simulink library "halin"  (R2021b)
settings: Solver=VariableStepAuto  StartTime=0.0  StopTime=10.0  RelTol=1e-3
undefined symbols (not defined in the file): TRUE
libraries: FVT_lib x100, hcu_lib x41
(part 1 of 10)
settings Model: Creator=13168  LastModifiedBy=FVT23010
settings SolverCC: AlgebraicLoopSolver=TrustRegion
settings DataIOCC: SaveFormat=Array  SignalLoggingSaveFormat=ModelDataLogs  ReturnWorkspaceOutputs=off
settings OptimizationCC: BlockReduction=off  BooleanDataType=off
settings DebuggingCC: SaveWithParameterizedLinksMsg=none  UnderspecifiedInitializationDetection=Classic  MergeDetectMultiDrivingBlocksExec=none  SignalResolutionControl=TryResolveAllWithWarning  SFMachineParentedDataDiag=warning
settings HardwareCC: TargetUnknown=on
settings ModelReferenceCC: PropagateSignalLabelsOutOfModel=off
settings ConfigComp: CovMetricSettings=dw  CovSaveCumulativeToWorkspaceVar=on  CovSaveSingleToWorkspaceVar=on

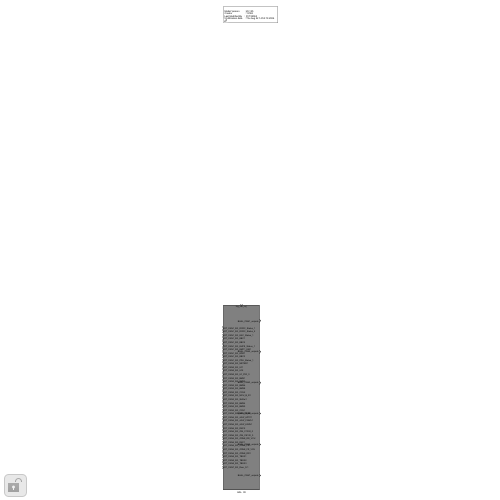
[thumbnail: Simulink's stored preview of the top-level diagram]
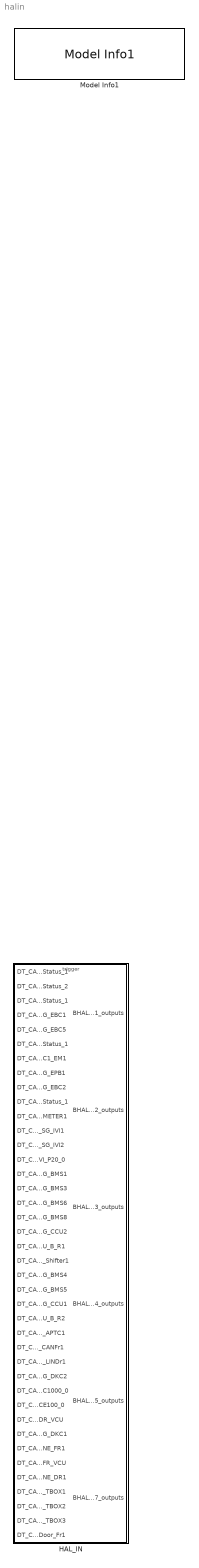
== system halin ==
  HAL_IN : Subsystem
      settings: RTWSystemCode=Nonreusable function  RTWFcnNameOpts=Use subsystem name  RTWFileNameOpts=Use subsystem name
  Model Info1 : hcu_lib/Model Info1  BlockCM=None  Frame=on  DisplayStringWithTags=|  HorizontalTextAlignment=Left  LeftAlignmentValue=0.02  SourceBlockDiagram=hcu_lib  TagMaxNumber=20
      | Model Version        : %<ModelVersion>
      | Creator                   : %<Creator>
      | Last Modified By    : %<LastModifiedBy>
      | Modification date    : %<LastModificationDate>
      settings: SourceProductName=HCU Relative Block Library

== system halin/HAL_IN ==
  DT_CAN1_SG_DCDC_Status_1 : Inport
  DT_CAN1_SG_DCDC_Status_2 : Inport  Port=2
  DT_CAN1_SG_EAC_Status_1 : Inport  Port=3
  DT_CAN1_SG_EBC1 : Inport  Port=4
  DT_CAN1_SG_EBC5 : Inport  Port=5
  DT_CAN1_SG_EHPS_Status_1 : Inport  Port=6
  DT_CAN1_SG_EMC1_EM1 : Inport  Port=7
  DT_CAN1_SG_EPB1 : Inport  Port=8
  DT_CAN1_SG_EBC2 : Inport  Port=9
  DT_CAN1_SG_PDU_Status_1 : Inport  Port=10
  DT_CAN2_SG_METER1 : Inport  Port=11
  DT_CAN2_SG_IVI1 : Inport  Port=12
  DT_CAN2_SG_IVI2 : Inport  Port=13
  DT_CAN2_SG_IVI_P20_0 : Inport  Port=14
  DT_CAN3_SG_BMS1 : Inport  Port=15
  DT_CAN3_SG_BMS3 : Inport  Port=16
  DT_CAN3_SG_BMS6 : Inport  Port=17
  DT_CAN3_SG_BMS8 : Inport  Port=18
  DT_CAN3_SG_CCU2 : Inport  Port=19
  DT_CAN3_SG_MCU_B_R1 : Inport  Port=20
  DT_CAN3_SG_Shifter1 : Inport  Port=21
  DT_CAN3_SG_BMS4 : Inport  Port=22
  DT_CAN3_SG_BMS5 : Inport  Port=23
  DT_CAN3_SG_CCU1 : Inport  Port=24
  DT_CAN3_SG_MCU_B_R2 : Inport  Port=25
  DT_CAN4_SG_zGW_APTC1 : Inport  Port=26
  DT_CAN4_SG_zGW_CANFr1 : Inport  Port=27
  DT_CAN4_SG_zGW_LINDr1 : Inport  Port=28
  DT_CAN4_SG_DKC2 : Inport  Port=29
  DT_CAN4_SG_Z24_C1000_0 : Inport  Port=30
  DT_CAN4_SG_Z24_CE100_0 : Inport  Port=31
  DT_CAN4_SG_ZONE_DR_VCU : Inport  Port=32
  DT_CAN4_SG_DKC1 : Inport  Port=33
  DT_CAN4_SG_ZONE_FR1 : Inport  Port=34
  DT_CAN4_SG_ZONE_FR_VCU : Inport  Port=35
  DT_CAN4_SG_ZONE_DR1 : Inport  Port=36
  DT_CAN5_SG_TBOX1 : Inport  Port=37
  DT_CAN5_SG_TBOX2 : Inport  Port=38
  DT_CAN5_SG_TBOX3 : Inport  Port=39
  DT_CAN7_SG_Door_Fr1 : Inport  Port=40
  trig_hal_in : TriggerPort  TriggerType=function-call  VariantControl=(inherit)
  CAN1 : Subsystem
  CAN2 : Subsystem
  CAN3 : Subsystem
  CAN4 : Subsystem
  CAN5 : Subsystem
  CAN7 : Subsystem
  BHAL_CAN1_outputs : Outport  OutDataTypeStr=Bus: BHAL_CAN1_outputs
  BHAL_CAN2_outputs : Outport  Port=2  OutDataTypeStr=Bus: BHAL_CAN2_outputs
  BHAL_CAN3_outputs : Outport  Port=3  OutDataTypeStr=Bus: BHAL_CAN3_outputs
  BHAL_CAN4_outputs : Outport  Port=4  OutDataTypeStr=Bus: BHAL_CAN4_outputs
  BHAL_CAN5_outputs : Outport  Port=5  OutDataTypeStr=Bus: BHAL_CAN5_outputs
  BHAL_CAN7_outputs : Outport  Port=6  OutDataTypeStr=Bus: BHAL_CAN7_outputs
  wires:
  DT_CAN5_SG_TBOX1/1 -> CAN5/1(DT_CAN5_SG_TBOX1)
  DT_CAN3_SG_CCU1/1 -> CAN3/10(DT_CAN3_SG_CCU1)
  DT_CAN3_SG_BMS5/1 -> CAN3/9(DT_CAN3_SG_BMS5)
  DT_CAN3_SG_BMS4/1 -> CAN3/8(DT_CAN3_SG_BMS4)
  DT_CAN3_SG_Shifter1/1 -> CAN3/7(DT_CAN3_SG_Shifter1)
  DT_CAN3_SG_MCU_B_R1/1 -> CAN3/6(DT_CAN3_SG_MCU_B_R1)
  DT_CAN3_SG_CCU2/1 -> CAN3/5(DT_CAN3_SG_CCU2)
  DT_CAN3_SG_BMS8/1 -> CAN3/4(DT_CAN3_SG_BMS8)
  CAN7/1(HAL_CAN7_outputs) -> BHAL_CAN7_outputs/1
  DT_CAN3_SG_BMS3/1 -> CAN3/2(DT_CAN3_SG_BMS3)
  DT_CAN3_SG_BMS1/1 -> CAN3/1(DT_CAN3_SG_BMS1)
  CAN1/1(HAL_CAN1_outputs) -> BHAL_CAN1_outputs/1
  CAN3/1(HAL_CAN3_outputs) -> BHAL_CAN3_outputs/1
  CAN4/1(HAL_CAN4_outputs) -> BHAL_CAN4_outputs/1
  DT_CAN1_SG_EMC1_EM1/1 -> CAN1/7(DT_CAN1_SG_EMC1_EM1)
  DT_CAN1_SG_EBC5/1 -> CAN1/5(DT_CAN1_SG_EBC5)
  DT_CAN1_SG_EHPS_Status_1/1 -> CAN1/6(DT_CAN1_SG_EHPS_Status_1)
  DT_CAN1_SG_EBC1/1 -> CAN1/4(DT_CAN1_SG_EBC1)
  DT_CAN1_SG_EAC_Status_1/1 -> CAN1/3(DT_CAN1_SG_EAC_Status_1)
  DT_CAN3_SG_BMS6/1 -> CAN3/3(DT_CAN3_SG_BMS6)
  DT_CAN1_SG_DCDC_Status_2/1 -> CAN1/2(DT_CAN1_SG_DCDC_Status_2)
  DT_CAN4_SG_ZONE_DR1/1 -> CAN4/11(DT_CAN4_SG_ZONE_DR1)
  DT_CAN1_SG_DCDC_Status_1/1 -> CAN1/1(DT_CAN1_SG_DCDC_Status_1)
  CAN2/1(HAL_CAN2_outputs) -> BHAL_CAN2_outputs/1
  DT_CAN3_SG_MCU_B_R2/1 -> CAN3/11(DT_CAN3_SG_MCU_B_R2)
  DT_CAN2_SG_IVI1/1 -> CAN2/2(DT_CAN2_SG_IVI1)
  DT_CAN5_SG_TBOX3/1 -> CAN5/3(DT_CAN5_SG_TBOX3)
  DT_CAN2_SG_METER1/1 -> CAN2/1(DT_CAN2_SG_METER1)
  DT_CAN1_SG_PDU_Status_1/1 -> CAN1/10(DT_CAN1_SG_PDU_Status_1)
  DT_CAN7_SG_Door_Fr1/1 -> CAN7/1(DT_CAN7_SG_Door_Fr1)
  DT_CAN1_SG_EPB1/1 -> CAN1/8(DT_CAN1_SG_EPB1)
  DT_CAN1_SG_EBC2/1 -> CAN1/9(DT_CAN1_SG_EBC2)
  DT_CAN2_SG_IVI2/1 -> CAN2/3(DT_CAN2_SG_IVI2)
  DT_CAN5_SG_TBOX2/1 -> CAN5/2(DT_CAN5_SG_TBOX2)
  DT_CAN2_SG_IVI_P20_0/1 -> CAN2/4(DT_CAN2_SG_IVI_P20_0)
  CAN5/1(HAL_CAN5_outputs) -> BHAL_CAN5_outputs/1
  DT_CAN4_SG_DKC1/1 -> CAN4/1(DT_CAN4_SG_DKC1)
  DT_CAN4_SG_ZONE_DR_VCU/1 -> CAN4/2(DT_CAN4_SG_ZONE_DR_VCU)
  DT_CAN4_SG_ZONE_FR1/1 -> CAN4/3(DT_CAN4_SG_ZONE_FR1)
  DT_CAN4_SG_ZONE_FR_VCU/1 -> CAN4/4(DT_CAN4_SG_ZONE_FR_VCU)
  DT_CAN4_SG_zGW_APTC1/1 -> CAN4/5(DT_CAN4_SG_zGW_APTC1)
  DT_CAN4_SG_zGW_LINDr1/1 -> CAN4/7(DT_CAN4_SG_zGW_LINDr1)
  DT_CAN4_SG_DKC2/1 -> CAN4/8(DT_CAN4_SG_DKC2)
  DT_CAN4_SG_Z24_C1000_0/1 -> CAN4/9(DT_CAN4_SG_Z24_C1000_0)
  DT_CAN4_SG_Z24_CE100_0/1 -> CAN4/10(DT_CAN4_SG_Z24_CE100_0)
  DT_CAN4_SG_zGW_CANFr1/1 -> CAN4/6(DT_CAN4_SG_zGW_CANFr1)

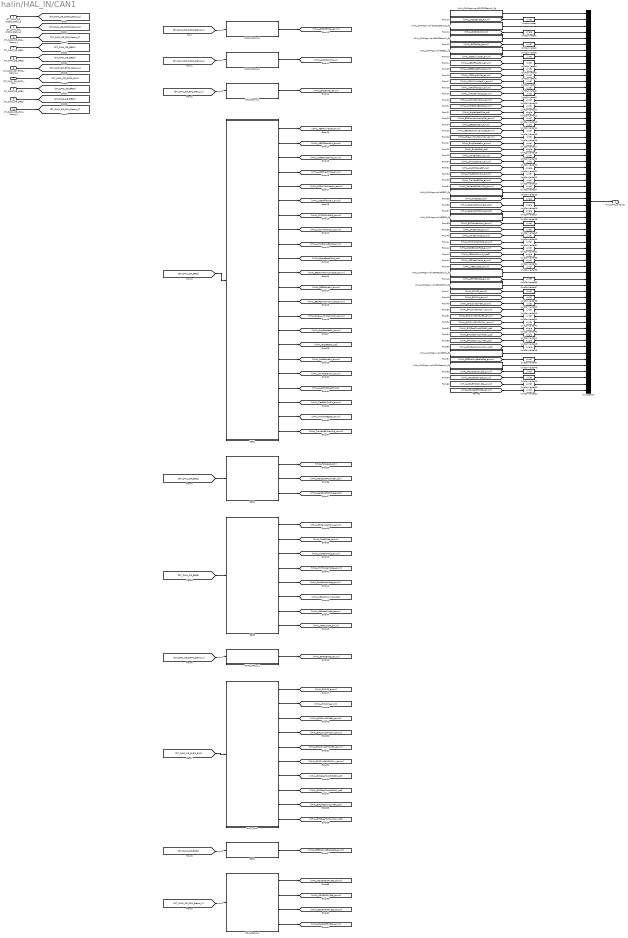
== system halin/HAL_IN/CAN1 ==
  DT_CAN1_SG_DCDC_Status_1 : Inport
  DT_CAN1_SG_DCDC_Status_2 : Inport  Port=2
  DT_CAN1_SG_EAC_Status_1 : Inport  Port=3
  DT_CAN1_SG_EBC1 : Inport  Port=4
  DT_CAN1_SG_EBC5 : Inport  Port=5
  DT_CAN1_SG_EHPS_Status_1 : Inport  Port=6
  DT_CAN1_SG_EMC1_EM1 : Inport  Port=7
  DT_CAN1_SG_EPB1 : Inport  Port=8
  DT_CAN1_SG_EBC2 : Inport  Port=9
  DT_CAN1_SG_PDU_Status_1 : Inport  Port=10
  DCDC_Status_1 : Subsystem
  DCDC_Status_2 : Subsystem
  EAC_Status_1 : Subsystem
  EBC1 : Subsystem
  EBC2 : Subsystem
  EBC5 : Subsystem
  EHPS_Status_1 : Subsystem
  EMC1_EM1 : Subsystem
  EPB1 : Subsystem
  PDU_Status_1 : Subsystem
  UnitConverter{,2..11,13..17,19..20,22..24,28..32,34..42,47..51} (40 alike) : DataTypeConversion  OutDataTypeStr=uint8
  UnitConverter{1,12,18,21,25..27,33,43..46} (12 alike) : DataTypeConversion  OutDataTypeStr=single
  VHAL_CANMsgInvalidDCDCStatus1_flg : Subsystem  AncestorBlock=FVT_lib/hal/MsgTimeoutJudge_CAN_AUTOSAR
      mask help: MeasumentTrigerEvent
      mask Display: fprintf('MsgTimeoutJudge_CAN\nAUTOSAR');
  VHAL_CANMsgInvalidDCDCStatus2_flg : Subsystem  AncestorBlock=FVT_lib/hal/MsgTimeoutJudge_CAN_AUTOSAR
      mask help: MeasumentTrigerEvent
      mask Display: fprintf('MsgTimeoutJudge_CAN\nAUTOSAR');
  VHAL_CANMsgInvalidEACStatus1_flg : Subsystem  AncestorBlock=FVT_lib/hal/MsgTimeoutJudge_CAN_AUTOSAR
      mask help: MeasumentTrigerEvent
      mask Display: fprintf('MsgTimeoutJudge_CAN\nAUTOSAR');
  VHAL_CANMsgInvalidEBC1_flg : Subsystem  AncestorBlock=FVT_lib/hal/MsgTimeoutJudge_CAN_AUTOSAR
      mask help: MeasumentTrigerEvent
      mask Display: fprintf('MsgTimeoutJudge_CAN\nAUTOSAR');
  VHAL_CANMsgInvalidEBC2_flg : Subsystem  AncestorBlock=FVT_lib/hal/MsgTimeoutJudge_CAN_AUTOSAR
      mask help: MeasumentTrigerEvent
      mask Display: fprintf('MsgTimeoutJudge_CAN\nAUTOSAR');
  VHAL_CANMsgInvalidEBC5_flg : Subsystem  AncestorBlock=FVT_lib/hal/MsgTimeoutJudge_CAN_AUTOSAR
      mask help: MeasumentTrigerEvent
      mask Display: fprintf('MsgTimeoutJudge_CAN\nAUTOSAR');
  VHAL_CANMsgInvalidEHPSStatus1_flg : Subsystem  AncestorBlock=FVT_lib/hal/MsgTimeoutJudge_CAN_AUTOSAR
      mask help: MeasumentTrigerEvent
      mask Display: fprintf('MsgTimeoutJudge_CAN\nAUTOSAR');
  VHAL_CANMsgInvalidEMC1EM1_flg : Subsystem  AncestorBlock=FVT_lib/hal/MsgTimeoutJudge_CAN_AUTOSAR
      mask help: MeasumentTrigerEvent
      mask Display: fprintf('MsgTimeoutJudge_CAN\nAUTOSAR');
  VHAL_CANMsgInvalidEPB1_flg : Subsystem  AncestorBlock=FVT_lib/hal/MsgTimeoutJudge_CAN_AUTOSAR
      mask help: MeasumentTrigerEvent
      mask Display: fprintf('MsgTimeoutJudge_CAN\nAUTOSAR');
  VHAL_CANMsgInvalidPDUStatus1_flg : Subsystem  AncestorBlock=FVT_lib/hal/MsgTimeoutJudge_CAN_AUTOSAR
      mask help: MeasumentTrigerEvent
      mask Display: fprintf('MsgTimeoutJudge_CAN\nAUTOSAR');
  bus_creator : BusCreator  Inputs=62
  HAL_CAN1_outputs : Outport
  wires:
  DT_CAN1_SG_DCDC_Status_1/1 -> [DT_CAN1_SG_DCDC_Status_1]
  DT_CAN1_SG_DCDC_Status_2/1 -> [DT_CAN1_SG_DCDC_Status_2]
  DT_CAN1_SG_EAC_Status_1/1 -> [DT_CAN1_SG_EAC_Status_1]
  DT_CAN1_SG_EBC1/1 -> [DT_CAN1_SG_EBC1]
  DT_CAN1_SG_EBC5/1 -> [DT_CAN1_SG_EBC5]
  DT_CAN1_SG_EHPS_Status_1/1 -> [DT_CAN1_SG_EHPS_Status_1]
  DT_CAN1_SG_EMC1_EM1/1 -> [DT_CAN1_SG_EMC1_EM1]
  DT_CAN1_SG_EPB1/1 -> [DT_CAN1_SG_EPB1]
  DT_CAN1_SG_EBC2/1 -> [DT_CAN1_SG_EBC2]
  DT_CAN1_SG_PDU_Status_1/1 -> [DT_CAN1_SG_PDU_Status_1]
  [DT_CAN1_SG_DCDC_Status_1] -> DCDC_Status_1/1(DT_CAN1_SG_DCDC_Status_1)
  [DT_CAN1_SG_DCDC_Status_2] -> DCDC_Status_2/1(DT_CAN1_SG_DCDC_Status_2)
  [DT_CAN1_SG_EAC_Status_1] -> EAC_Status_1/1(DT_CAN1_SG_EAC_Status_1)
  [DT_CAN1_SG_EBC1] -> EBC1/1(DT_CAN1_SG_EBC1)
  [DT_CAN1_SG_EBC2] -> EBC2/1(DT_CAN1_SG_EBC2)
  [DT_CAN1_SG_EBC5] -> EBC5/1(DT_CAN1_SG_EBC5)
  [DT_CAN1_SG_EHPS_Status_1] -> EHPS_Status_1/1(DT_CAN1_SG_EHPS_Status_1)
  [DT_CAN1_SG_EMC1_EM1] -> EMC1_EM1/1(DT_CAN1_SG_EMC1_EM1)
  [DT_CAN1_SG_EPB1] -> EPB1/1(DT_CAN1_SG_EPB1)
  [DT_CAN1_SG_PDU_Status_1] -> PDU_Status_1/1(DT_CAN1_SG_PDU_Status_1)
  bus_creator/1 -> HAL_CAN1_outputs/1
  VHAL_CANMsgInvalidDCDCStatus1_flg/1(Out) -> bus_creator/1
  DCDC_Status_1/1(VHAL_DCDCEnSta_enum) -> [VHAL_DCDCEnSta_enum]
  UnitConverter/1 -> bus_creator/2  "VHAL_DCDCEnSta_enum"
  [VHAL_DCDCEnSta_enum] -> UnitConverter/1
  VHAL_CANMsgInvalidDCDCStatus2_flg/1(Out) -> bus_creator/3
  DCDC_Status_2/1(VHAL_DCDCOutVol_V) -> [VHAL_DCDCOutVol_V]
  UnitConverter1/1 -> bus_creator/4  "VHAL_DCDCOutVol_V"
  [VHAL_DCDCOutVol_V] -> UnitConverter1/1
  VHAL_CANMsgInvalidEACStatus1_flg/1(Out) -> bus_creator/5
  EAC_Status_1/1(VHAL_EACEnSta_enum) -> [VHAL_EACEnSta_enum]
  UnitConverter2/1 -> bus_creator/6  "VHAL_EACEnSta_enum"
  [VHAL_EACEnSta_enum] -> UnitConverter2/1
  VHAL_CANMsgInvalidEBC1_flg/1(Out) -> bus_creator/7
  EBC1/1(VHAL_ABSFullyOper_enum) -> [VHAL_ABSFullyOper_enum]
  UnitConverter3/1 -> bus_creator/8  "VHAL_ABSFullyOper_enum"
  [VHAL_ABSFullyOper_enum] -> UnitConverter3/1
  EBC1/2(VHAL_ABSOffroadSw_enum) -> [VHAL_ABSOffroadSw_enum]
  UnitConverter4/1 -> bus_creator/9  "VHAL_ABSOffroadSw_enum"
  [VHAL_ABSOffroadSw_enum] -> UnitConverter4/1
  EBC1/3(VHAL_ASRBrakeCtrlAtc_enum) -> [VHAL_ASRBrakeCtrlAtc_enum]
  UnitConverter5/1 -> bus_creator/10  "VHAL_ASRBrakeCtrlAtc_enum"
  [VHAL_ASRBrakeCtrlAtc_enum] -> UnitConverter5/1
  EBC1/4(VHAL_ASREngCtrlAtc_enum) -> [VHAL_ASREngCtrlAtc_enum]
  UnitConverter6/1 -> bus_creator/11  "VHAL_ASREngCtrlAtc_enum"
  [VHAL_ASREngCtrlAtc_enum] -> UnitConverter6/1
  EBC1/5(VHAL_ASRHillHolderSw_enum) -> [VHAL_ASRHillHolderSw_enum]
  UnitConverter7/1 -> bus_creator/12  "VHAL_ASRHillHolderSw_enum"
  [VHAL_ASRHillHolderSw_enum] -> UnitConverter7/1
  EBC1/6(VHAL_ASROffroadSw_enum) -> [VHAL_ASROffroadSw_enum]
  UnitConverter8/1 -> bus_creator/13  "VHAL_ASROffroadSw_enum"
  [VHAL_ASROffroadSw_enum] -> UnitConverter8/1
  EBC1/7(VHAL_ATCASRInfoSig_enum) -> [VHAL_ATCASRInfoSig_enum]
  UnitConverter9/1 -> bus_creator/14  "VHAL_ATCASRInfoSig_enum"
  [VHAL_ATCASRInfoSig_enum] -> UnitConverter9/1
  EBC1/8(VHAL_AcltrInterlockSw_enum) -> [VHAL_AcltrInterlockSw_enum]
  UnitConverter10/1 -> bus_creator/15  "VHAL_AcltrInterlockSw_enum"
  [VHAL_AcltrInterlockSw_enum] -> UnitConverter10/1
  EBC1/9(VHAL_AntiLBrakABSAct_enum) -> [VHAL_AntiLBrakABSAct_enum]
  UnitConverter11/1 -> bus_creator/16  "VHAL_AntiLBrakABSAct_enum"
  [VHAL_AntiLBrakABSAct_enum] -> UnitConverter11/1
  EBC1/10(VHAL_BrakePedalPos_pct) -> [VHAL_BrakePedalPos_pct]
  UnitConverter12/1 -> bus_creator/17  "VHAL_BrakePedalPos_pct"
  [VHAL_BrakePedalPos_pct] -> UnitConverter12/1
  EBC1/11(VHAL_EBSAmWarnLampSta_enum) -> [VHAL_EBSAmWarnLampSta_enum]
  UnitConverter13/1 -> bus_creator/18  "VHAL_EBSAmWarnLampSta_enum"
  [VHAL_EBSAmWarnLampSta_enum] -> UnitConverter13/1
  EBC1/12(VHAL_EBSBrakeSw_enum) -> [VHAL_EBSBrakeSw_enum]
  UnitConverter14/1 -> bus_creator/19  "VHAL_EBSBrakeSw_enum"
  [VHAL_EBSBrakeSw_enum] -> UnitConverter14/1
  EBC1/13(VHAL_EBSRedWarnLampSta_enum) -> [VHAL_EBSRedWarnLampSta_enum]
  UnitConverter15/1 -> bus_creator/20  "VHAL_EBSRedWarnLampSta_enum"
  [VHAL_EBSRedWarnLampSta_enum] -> UnitConverter15/1
  EBC1/14(VHAL_EngAuxShutdownSw_enum) -> [VHAL_EngAuxShutdownSw_enum]
  UnitConverter16/1 -> bus_creator/21  "VHAL_EngAuxShutdownSw_enum"
  [VHAL_EngAuxShutdownSw_enum] -> UnitConverter16/1
  EBC1/15(VHAL_EngDerateSw_enum) -> [VHAL_EngDerateSw_enum]
  UnitConverter17/1 -> bus_creator/22  "VHAL_EngDerateSw_enum"
  [VHAL_EngDerateSw_enum] -> UnitConverter17/1
  EBC1/16(VHAL_EngRetSel_pct) -> [VHAL_EngRetSel_pct]
  UnitConverter18/1 -> bus_creator/23  "VHAL_EngRetSel_pct"
  [VHAL_EngRetSel_pct] -> UnitConverter18/1
  EBC1/17(VHAL_HaltBrakeSw_enum) -> [VHAL_HaltBrakeSw_enum]
  UnitConverter19/1 -> bus_creator/24  "VHAL_HaltBrakeSw_enum"
  [VHAL_HaltBrakeSw_enum] -> UnitConverter19/1
  EBC1/18(VHAL_RmAccelEnSw_enum) -> [VHAL_RmAccelEnSw_enum]
  UnitConverter20/1 -> bus_creator/25  "VHAL_RmAccelEnSw_enum"
  [VHAL_RmAccelEnSw_enum] -> UnitConverter20/1
  EBC1/19(VHAL_SACtrlBrakeCtrl_SA) -> [VHAL_SACtrlBrakeCtrl_SA]
  UnitConverter21/1 -> bus_creator/26  "VHAL_SACtrlBrakeCtrl_SA"
  [VHAL_SACtrlBrakeCtrl_SA] -> UnitConverter21/1
  EBC1/20(VHAL_TractCtrlOvrSw_enum) -> [VHAL_TractCtrlOvrSw_enum]
  UnitConverter22/1 -> bus_creator/27  "VHAL_TractCtrlOvrSw_enum"
  [VHAL_TractCtrlOvrSw_enum] -> UnitConverter22/1
  EBC1/21(VHAL_TrailerABSSta_enum) -> [VHAL_TrailerABSSta_enum]
  UnitConverter23/1 -> bus_creator/28  "VHAL_TrailerABSSta_enum"
  [VHAL_TrailerABSSta_enum] -> UnitConverter23/1
  EBC1/22(VHAL_TrailerABSWarnSig_enum) -> [VHAL_TrailerABSWarnSig_enum]
  UnitConverter24/1 -> bus_creator/29  "VHAL_TrailerABSWarnSig_enum"
  [VHAL_TrailerABSWarnSig_enum] -> UnitConverter24/1
  VHAL_CANMsgInvalidEBC2_flg/1(Out) -> bus_creator/30
  EBC2/1(VHAL_FASpeed_kph) -> [VHAL_FASpeed_kph]
  UnitConverter25/1 -> bus_creator/31  "VHAL_FASpeed_kph"
  [VHAL_FASpeed_kph] -> UnitConverter25/1
  EBC2/2(VHAL_RelaSpdFALWheel_kph) -> [VHAL_RelaSpdFALWheel_kph]
  UnitConverter26/1 -> bus_creator/32  "VHAL_RelaSpdFALWheel_kph"
  [VHAL_RelaSpdFALWheel_kph] -> UnitConverter26/1
  EBC2/3(VHAL_RelaSpdFARWheel_kph) -> [VHAL_RelaSpdFARWheel_kph]
  UnitConverter27/1 -> bus_creator/33  "VHAL_RelaSpdFARWheel_kph"
  [VHAL_RelaSpdFARWheel_kph] -> UnitConverter27/1
  VHAL_CANMsgInvalidEBC5_flg/1(Out) -> bus_creator/34
  EBC5/1(VHAL_BrkTempeWarn_enum) -> [VHAL_BrkTempeWarn_enum]
  UnitConverter28/1 -> bus_creator/35  "VHAL_BrkTempeWarn_enum"
  [VHAL_BrkTempeWarn_enum] -> UnitConverter28/1
  EBC5/2(VHAL_FndBrkUse_enum) -> [VHAL_FndBrkUse_enum]
  UnitConverter29/1 -> bus_creator/36  "VHAL_FndBrkUse_enum"
  [VHAL_FndBrkUse_enum] -> UnitConverter29/1
  EBC5/3(VHAL_HaltBrkMode_enum) -> [VHAL_HaltBrkMode_enum]
  UnitConverter30/1 -> bus_creator/37  "VHAL_HaltBrkMode_enum"
  [VHAL_HaltBrkMode_enum] -> UnitConverter30/1
  EBC5/4(VHAL_HillHolderMode_enum) -> [VHAL_HillHolderMode_enum]
  UnitConverter31/1 -> bus_creator/38  "VHAL_HillHolderMode_enum"
  [VHAL_HillHolderMode_enum] -> UnitConverter31/1
  EBC5/5(VHAL_ParkBrkActuFAct_enum) -> [VHAL_ParkBrkActuFAct_enum]
  UnitConverter32/1 -> bus_creator/39  "VHAL_ParkBrkActuFAct_enum"
  [VHAL_ParkBrkActuFAct_enum] -> UnitConverter32/1
  EBC5/6(VHAL_XBRAcltnLimit_mps2) -> [VHAL_XBRAcltnLimit_mps2]
  UnitConverter33/1 -> bus_creator/40  "VHAL_XBRAcltnLimit_mps2"
  [VHAL_XBRAcltnLimit_mps2] -> UnitConverter33/1
  EBC5/7(VHAL_XBRActtrlMode_enum) -> [VHAL_XBRActtrlMode_enum]
  UnitConverter34/1 -> bus_creator/41  "VHAL_XBRActtrlMode_enum"
  [VHAL_XBRActtrlMode_enum] -> UnitConverter34/1
  EBC5/8(VHAL_XBRSysSta_enum) -> [VHAL_XBRSysSta_enum]
  UnitConverter35/1 -> bus_creator/42  "VHAL_XBRSysSta_enum"
  [VHAL_XBRSysSta_enum] -> UnitConverter35/1
  VHAL_CANMsgInvalidEHPSStatus1_flg/1(Out) -> bus_creator/43
  EHPS_Status_1/1(VHAL_EHPSEnSta_enum) -> [VHAL_EHPSEnSta_enum]
  UnitConverter36/1 -> bus_creator/44  "VHAL_EHPSEnSta_enum"
  [VHAL_EHPSEnSta_enum] -> UnitConverter36/1
  VHAL_CANMsgInvalidEMC1EM1_flg/1(Out) -> bus_creator/45
  EMC1_EM1/1(VHAL_EM1CS_enum) -> [VHAL_EM1CS_enum]
  UnitConverter37/1 -> bus_creator/46  "VHAL_EM1CS_enum"
  [VHAL_EM1CS_enum] -> UnitConverter37/1
  EMC1_EM1/2(VHAL_EM1Cnt_enum) -> [VHAL_EM1Cnt_enum]
  UnitConverter38/1 -> bus_creator/47  "VHAL_EM1Cnt_enum"
  [VHAL_EM1Cnt_enum] -> UnitConverter38/1
  EMC1_EM1/3(VHAL_EM1OvrCtrlMBrk_enum) -> [VHAL_EM1OvrCtrlMBrk_enum]
  UnitConverter39/1 -> bus_creator/48  "VHAL_EM1OvrCtrlMBrk_enum"
  [VHAL_EM1OvrCtrlMBrk_enum] -> UnitConverter39/1
  EMC1_EM1/4(VHAL_EM1OvrCtrlMDriv_enum) -> [VHAL_EM1OvrCtrlMDriv_enum]
  UnitConverter40/1 -> bus_creator/49  "VHAL_EM1OvrCtrlMDriv_enum"
  [VHAL_EM1OvrCtrlMDriv_enum] -> UnitConverter40/1
  EMC1_EM1/5(VHAL_EM1OvrCtrlMPriBrk_enum) -> [VHAL_EM1OvrCtrlMPriBrk_enum]
  UnitConverter41/1 -> bus_creator/50  "VHAL_EM1OvrCtrlMPriBrk_enum"
  [VHAL_EM1OvrCtrlMPriBrk_enum] -> UnitConverter41/1
  EMC1_EM1/6(VHAL_EM1OvrCtrlMPriDriv_enum) -> [VHAL_EM1OvrCtrlMPriDriv_enum]
  UnitConverter42/1 -> bus_creator/51  "VHAL_EM1OvrCtrlMPriDriv_enum"
  [VHAL_EM1OvrCtrlMPriDriv_enum] -> UnitConverter42/1
  EMC1_EM1/7(VHAL_EM1ReqTorqHRlsBrk_pct) -> [VHAL_EM1ReqTorqHRlsBrk_pct]
  UnitConverter43/1 -> bus_creator/52  "VHAL_EM1ReqTorqHRlsBrk_pct"
  [VHAL_EM1ReqTorqHRlsBrk_pct] -> UnitConverter43/1
  EMC1_EM1/8(VHAL_EM1ReqTorqHRlsDri_pct) -> [VHAL_EM1ReqTorqHRlsDri_pct]
  UnitConverter44/1 -> bus_creator/53  "VHAL_EM1ReqTorqHRlsDri_pct"
  [VHAL_EM1ReqTorqHRlsDri_pct] -> UnitConverter44/1
  EMC1_EM1/9(VHAL_EM1ReqTorqLimBrk_pct) -> [VHAL_EM1ReqTorqLimBrk_pct]
  UnitConverter45/1 -> bus_creator/54  "VHAL_EM1ReqTorqLimBrk_pct"
  [VHAL_EM1ReqTorqLimBrk_pct] -> UnitConverter45/1
  EMC1_EM1/10(VHAL_EM1ReqTorqLimDriv_pct) -> [VHAL_EM1ReqTorqLimDriv_pct]
  UnitConverter46/1 -> bus_creator/55  "VHAL_EM1ReqTorqLimDriv_pct"
  [VHAL_EM1ReqTorqLimDriv_pct] -> UnitConverter46/1
  VHAL_CANMsgInvalidEPB1_flg/1(Out) -> bus_creator/56
  EPB1/1(VHAL_EPBParkingBrakeSta_enum) -> [VHAL_EPBParkingBrakeSta_enum]
  UnitConverter47/1 -> bus_creator/57  "VHAL_EPBParkingBrakeSta_enum"
  [VHAL_EPBParkingBrakeSta_enum] -> UnitConverter47/1
  VHAL_CANMsgInvalidPDUStatus1_flg/1(Out) -> bus_creator/58
  PDU_Status_1/1(VHAL_PDUDCDCRlySta_enum) -> [VHAL_PDUDCDCRlySta_enum]
  UnitConverter48/1 -> bus_creator/59  "VHAL_PDUDCDCRlySta_enum"
  [VHAL_PDUDCDCRlySta_enum] -> UnitConverter48/1
  PDU_Status_1/2(VHAL_PDUEACRlySta_enum) -> [VHAL_PDUEACRlySta_enum]
  UnitConverter49/1 -> bus_creator/60  "VHAL_PDUEACRlySta_enum"
  [VHAL_PDUEACRlySta_enum] -> UnitConverter49/1
  PDU_Status_1/3(VHAL_PDUEHPSRlySta_enum) -> [VHAL_PDUEHPSRlySta_enum]
  UnitConverter50/1 -> bus_creator/61  "VHAL_PDUEHPSRlySta_enum"
  [VHAL_PDUEHPSRlySta_enum] -> UnitConverter50/1
  PDU_Status_1/4(VHAL_PDUSelfChkSta_enum) -> [VHAL_PDUSelfChkSta_enum]
  UnitConverter51/1 -> bus_creator/62  "VHAL_PDUSelfChkSta_enum"
  [VHAL_PDUSelfChkSta_enum] -> UnitConverter51/1

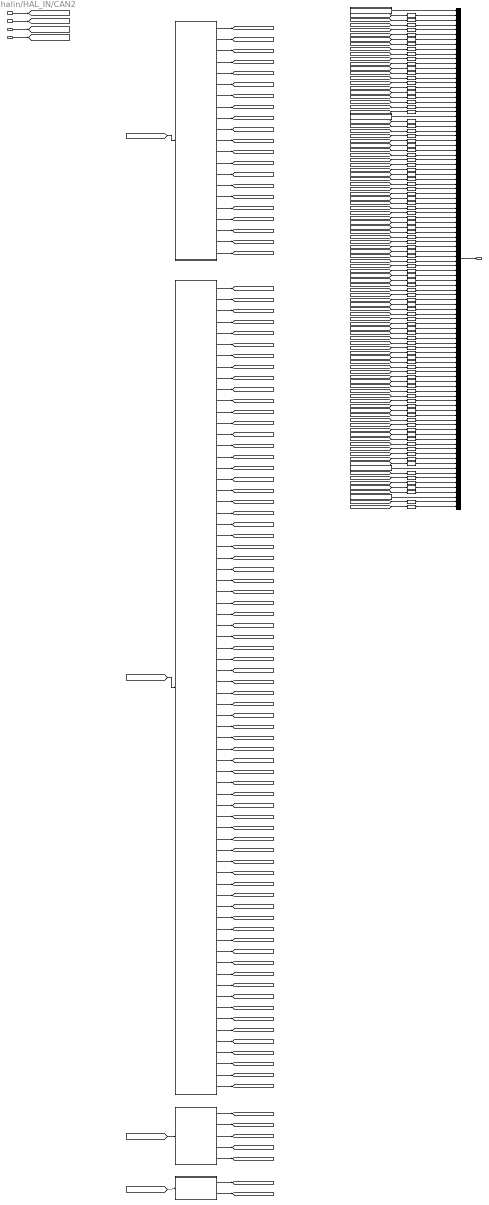
== system halin/HAL_IN/CAN2 ==
  DT_CAN2_SG_METER1 : Inport
  DT_CAN2_SG_IVI1 : Inport  Port=2
  DT_CAN2_SG_IVI2 : Inport  Port=3
  DT_CAN2_SG_IVI_P20_0 : Inport  Port=4
  IVI1 : Subsystem
  IVI2 : Subsystem
  IVI_P20_0 : Subsystem
  METER1 : Subsystem
  UnitConverter{,1,3..9,17..20,22..23,28..31,33,36,41,44,47..48,51..56,61..62,67,69..70,73..75,77,79,81..82,84,87..90,93..95,97} (52 alike) : DataTypeConversion  OutDataTypeStr=boolean
  UnitConverter{2,10,24..27,32,34..35,39..40,42..43,45..46,49..50,64..66,68,78,80,83,85..86,96} (27 alike) : DataTypeConversion  OutDataTypeStr=uint8
  UnitConverter{11..16,21,37,57..60,63,71..72,76,91..92,98..99} (20 alike) : DataTypeConversion  OutDataTypeStr=single
  UnitConverter38 : DataTypeConversion  OutDataTypeStr=uint32
  VHAL_CANMsgInvalidIVI1_flg : Subsystem  AncestorBlock=FVT_lib/hal/MsgTimeoutJudge_CAN_AUTOSAR
      mask help: MeasumentTrigerEvent
      mask Display: fprintf('MsgTimeoutJudge_CAN\nAUTOSAR');
  VHAL_CANMsgInvalidIVI2_flg : Subsystem  AncestorBlock=FVT_lib/hal/MsgTimeoutJudge_CAN_AUTOSAR
      mask help: MeasumentTrigerEvent
      mask Display: fprintf('MsgTimeoutJudge_CAN\nAUTOSAR');
  VHAL_CANMsgInvalidIVIP200_flg : Subsystem  AncestorBlock=FVT_lib/hal/MsgTimeoutJudge_CAN_AUTOSAR
      mask help: MeasumentTrigerEvent
      mask Display: fprintf('MsgTimeoutJudge_CAN\nAUTOSAR');
  VHAL_CANMsgInvalidMETER1_flg : Subsystem  AncestorBlock=FVT_lib/hal/MsgTimeoutJudge_CAN_AUTOSAR
      mask help: MeasumentTrigerEvent
      mask Display: fprintf('MsgTimeoutJudge_CAN\nAUTOSAR');
  bus_creator : BusCreator  Inputs=104
  HAL_CAN2_outputs : Outport
  wires:
  DT_CAN2_SG_METER1/1 -> [DT_CAN2_SG_METER1]
  DT_CAN2_SG_IVI1/1 -> [DT_CAN2_SG_IVI1]
  DT_CAN2_SG_IVI2/1 -> [DT_CAN2_SG_IVI2]
  DT_CAN2_SG_IVI_P20_0/1 -> [DT_CAN2_SG_IVI_P20_0]
  [DT_CAN2_SG_IVI1] -> IVI1/1(DT_CAN2_SG_IVI1)
  [DT_CAN2_SG_IVI2] -> IVI2/1(DT_CAN2_SG_IVI2)
  [DT_CAN2_SG_IVI_P20_0] -> IVI_P20_0/1(DT_CAN2_SG_IVI_P20_0)
  [DT_CAN2_SG_METER1] -> METER1/1(DT_CAN2_SG_METER1)
  bus_creator/1 -> HAL_CAN2_outputs/1
  VHAL_CANMsgInvalidIVI1_flg/1(Out) -> bus_creator/1
  IVI1/1(VHAL_AmbLighLowBatAlertSW_flg) -> [VHAL_AmbLighLowBatAlertSW_flg]
  UnitConverter/1 -> bus_creator/2  "VHAL_AmbLighLowBatAlertSW_flg"
  [VHAL_AmbLighLowBatAlertSW_flg] -> UnitConverter/1
  IVI1/2(VHAL_AmbLighSafetyAlertSW_flg) -> [VHAL_AmbLighSafetyAlertSW_flg]
  UnitConverter1/1 -> bus_creator/3  "VHAL_AmbLighSafetyAlertSW_flg"
  [VHAL_AmbLighSafetyAlertSW_flg] -> UnitConverter1/1
  IVI1/3(VHAL_AmbLightColorSet_enum) -> [VHAL_AmbLightColorSet_enum]
  UnitConverter2/1 -> bus_creator/4  "VHAL_AmbLightColorSet_enum"
  [VHAL_AmbLightColorSet_enum] -> UnitConverter2/1
  IVI1/4(VHAL_AmbLightDimInDarkSW_flg) -> [VHAL_AmbLightDimInDarkSW_flg]
  UnitConverter3/1 -> bus_creator/5  "VHAL_AmbLightDimInDarkSW_flg"
  [VHAL_AmbLightDimInDarkSW_flg] -> UnitConverter3/1
  IVI1/5(VHAL_AmbLightSW_flg) -> [VHAL_AmbLightSW_flg]
  UnitConverter4/1 -> bus_creator/6  "VHAL_AmbLightSW_flg"
  [VHAL_AmbLightSW_flg] -> UnitConverter4/1
  IVI1/6(VHAL_AmbLightWlcmLightSW_flg) -> [VHAL_AmbLightWlcmLightSW_flg]
  UnitConverter5/1 -> bus_creator/7  "VHAL_AmbLightWlcmLightSW_flg"
  [VHAL_AmbLightWlcmLightSW_flg] -> UnitConverter5/1
  IVI1/7(VHAL_FCPFrEvtBtnACMaxReq_flg) -> [VHAL_FCPFrEvtBtnACMaxReq_flg]
  UnitConverter6/1 -> bus_creator/8  "VHAL_FCPFrEvtBtnACMaxReq_flg"
  [VHAL_FCPFrEvtBtnACMaxReq_flg] -> UnitConverter6/1
  IVI1/8(VHAL_FCPFrEvtBtnACReq_flg) -> [VHAL_FCPFrEvtBtnACReq_flg]
  UnitConverter7/1 -> bus_creator/9  "VHAL_FCPFrEvtBtnACReq_flg"
  [VHAL_FCPFrEvtBtnACReq_flg] -> UnitConverter7/1
  IVI1/9(VHAL_FCPFrEvtBtnAutoReq_flg) -> [VHAL_FCPFrEvtBtnAutoReq_flg]
  UnitConverter8/1 -> bus_creator/10  "VHAL_FCPFrEvtBtnAutoReq_flg"
  [VHAL_FCPFrEvtBtnAutoReq_flg] -> UnitConverter8/1
  IVI1/10(VHAL_FCPFrEvtBtnSyncReq_flg) -> [VHAL_FCPFrEvtBtnSyncReq_flg]
  UnitConverter9/1 -> bus_creator/11  "VHAL_FCPFrEvtBtnSyncReq_flg"
  [VHAL_FCPFrEvtBtnSyncReq_flg] -> UnitConverter9/1
  IVI1/11(VHAL_IVITimeCheck_enum) -> [VHAL_IVITimeCheck_enum]
  UnitConverter10/1 -> bus_creator/12  "VHAL_IVITimeCheck_enum"
  [VHAL_IVITimeCheck_enum] -> UnitConverter10/1
  IVI1/12(VHAL_IVITimeDay_DAY) -> [VHAL_IVITimeDay_DAY]
  UnitConverter11/1 -> bus_creator/13  "VHAL_IVITimeDay_DAY"
  [VHAL_IVITimeDay_DAY] -> UnitConverter11/1
  IVI1/13(VHAL_IVITimeHour_hr) -> [VHAL_IVITimeHour_hr]
  UnitConverter12/1 -> bus_creator/14  "VHAL_IVITimeHour_hr"
  [VHAL_IVITimeHour_hr] -> UnitConverter12/1
  IVI1/14(VHAL_IVITimeMinute_min) -> [VHAL_IVITimeMinute_min]
  UnitConverter13/1 -> bus_creator/15  "VHAL_IVITimeMinute_min"
  [VHAL_IVITimeMinute_min] -> UnitConverter13/1
  IVI1/15(VHAL_IVITimeMonth_MONTH) -> [VHAL_IVITimeMonth_MONTH]
  UnitConverter14/1 -> bus_creator/16  "VHAL_IVITimeMonth_MONTH"
  [VHAL_IVITimeMonth_MONTH] -> UnitConverter14/1
  IVI1/16(VHAL_IVITimeSecond_s) -> [VHAL_IVITimeSecond_s]
  UnitConverter15/1 -> bus_creator/17  "VHAL_IVITimeSecond_s"
  [VHAL_IVITimeSecond_s] -> UnitConverter15/1
  IVI1/17(VHAL_IVITimeYear_YEAR) -> [VHAL_IVITimeYear_YEAR]
  UnitConverter16/1 -> bus_creator/18  "VHAL_IVITimeYear_YEAR"
  [VHAL_IVITimeYear_YEAR] -> UnitConverter16/1
  IVI1/18(VHAL_LINKtoDrive_flg) -> [VHAL_LINKtoDrive_flg]
  UnitConverter17/1 -> bus_creator/19  "VHAL_LINKtoDrive_flg"
  [VHAL_LINKtoDrive_flg] -> UnitConverter17/1
  IVI1/19(VHAL_OpenDrOpenWdoSW_flg) -> [VHAL_OpenDrOpenWdoSW_flg]
  UnitConverter18/1 -> bus_creator/20  "VHAL_OpenDrOpenWdoSW_flg"
  [VHAL_OpenDrOpenWdoSW_flg] -> UnitConverter18/1
  IVI1/20(VHAL_PWCONTINUEUSE_flg) -> [VHAL_PWCONTINUEUSE_flg]
  UnitConverter19/1 -> bus_creator/21  "VHAL_PWCONTINUEUSE_flg"
  [VHAL_PWCONTINUEUSE_flg] -> UnitConverter19/1
  IVI1/21(VHAL_SmartEcoModeSW_flg) -> [VHAL_SmartEcoModeSW_flg]
  UnitConverter20/1 -> bus_creator/22  "VHAL_SmartEcoModeSW_flg"
  [VHAL_SmartEcoModeSW_flg] -> UnitConverter20/1
  VHAL_CANMsgInvalidIVI2_flg/1(Out) -> bus_creator/23
  IVI2/1(VHAL_ACChgCurSet_A) -> [VHAL_ACChgCurSet_A]
  UnitConverter21/1 -> bus_creator/24  "VHAL_ACChgCurSet_A"
  [VHAL_ACChgCurSet_A] -> UnitConverter21/1
  IVI2/2(VHAL_AVMErrSTA_flg) -> [VHAL_AVMErrSTA_flg]
  UnitConverter22/1 -> bus_creator/25  "VHAL_AVMErrSTA_flg"
  [VHAL_AVMErrSTA_flg] -> UnitConverter22/1
  IVI2/3(VHAL_AVMOFFRecButt_flg) -> [VHAL_AVMOFFRecButt_flg]
  UnitConverter23/1 -> bus_creator/26  "VHAL_AVMOFFRecButt_flg"
  [VHAL_AVMOFFRecButt_flg] -> UnitConverter23/1
  IVI2/4(VHAL_AVMParkingmode_enum) -> [VHAL_AVMParkingmode_enum]
  UnitConverter24/1 -> bus_creator/27  "VHAL_AVMParkingmode_enum"
  [VHAL_AVMParkingmode_enum] -> UnitConverter24/1
  IVI2/5(VHAL_AVMparkingcancel_enum) -> [VHAL_AVMparkingcancel_enum]
  UnitConverter25/1 -> bus_creator/28  "VHAL_AVMparkingcancel_enum"
  [VHAL_AVMparkingcancel_enum] -> UnitConverter25/1
  IVI2/6(VHAL_AVMparkingexcute_enum) -> [VHAL_AVMparkingexcute_enum]
  UnitConverter26/1 -> bus_creator/29  "VHAL_AVMparkingexcute_enum"
  [VHAL_AVMparkingexcute_enum] -> UnitConverter26/1
  IVI2/7(VHAL_CAASSw_enum) -> [VHAL_CAASSw_enum]
  UnitConverter27/1 -> bus_creator/30  "VHAL_CAASSw_enum"
  [VHAL_CAASSw_enum] -> UnitConverter27/1
  IVI2/8(VHAL_CDLLockButt_flg) -> [VHAL_CDLLockButt_flg]
  UnitConverter28/1 -> bus_creator/31  "VHAL_CDLLockButt_flg"
  [VHAL_CDLLockButt_flg] -> UnitConverter28/1
  IVI2/9(VHAL_CDLUnlockButt_flg) -> [VHAL_CDLUnlockButt_flg]
  UnitConverter29/1 -> bus_creator/32  "VHAL_CDLUnlockButt_flg"
  [VHAL_CDLUnlockButt_flg] -> UnitConverter29/1
  IVI2/10(VHAL_DSEATantiset_flg) -> [VHAL_DSEATantiset_flg]
  UnitConverter30/1 -> bus_creator/33  "VHAL_DSEATantiset_flg"
  [VHAL_DSEATantiset_flg] -> UnitConverter30/1
  IVI2/11(VHAL_DSEATentryfunset_flg) -> [VHAL_DSEATentryfunset_flg]
  UnitConverter31/1 -> bus_creator/34  "VHAL_DSEATentryfunset_flg"
  [VHAL_DSEATentryfunset_flg] -> UnitConverter31/1
  IVI2/12(VHAL_DSEATventreq_enum) -> [VHAL_DSEATventreq_enum]
  UnitConverter32/1 -> bus_creator/35  "VHAL_DSEATventreq_enum"
  [VHAL_DSEATventreq_enum] -> UnitConverter32/1
  IVI2/13(VHAL_Distanceunit_flg) -> [VHAL_Distanceunit_flg]
  UnitConverter33/1 -> bus_creator/36  "VHAL_Distanceunit_flg"
  [VHAL_Distanceunit_flg] -> UnitConverter33/1
  IVI2/14(VHAL_ESCSWCmd_enum) -> [VHAL_ESCSWCmd_enum]
  UnitConverter34/1 -> bus_creator/37  "VHAL_ESCSWCmd_enum"
  [VHAL_ESCSWCmd_enum] -> UnitConverter34/1
  IVI2/15(VHAL_FSOffSw_enum) -> [VHAL_FSOffSw_enum]
  UnitConverter35/1 -> bus_creator/38  "VHAL_FSOffSw_enum"
  [VHAL_FSOffSw_enum] -> UnitConverter35/1
  IVI2/16(VHAL_FollowMeSW_flg) -> [VHAL_FollowMeSW_flg]
  UnitConverter36/1 -> bus_creator/39  "VHAL_FollowMeSW_flg"
  [VHAL_FollowMeSW_flg] -> UnitConverter36/1
  IVI2/17(VHAL_GPSLAT_s) -> [VHAL_GPSLAT_s]
  UnitConverter37/1 -> bus_creator/40  "VHAL_GPSLAT_s"
  [VHAL_GPSLAT_s] -> UnitConverter37/1
  IVI2/18(VHAL_GPSLONG_enum) -> [VHAL_GPSLONG_enum]
  UnitConverter38/1 -> bus_creator/41  "VHAL_GPSLONG_enum"
  [VHAL_GPSLONG_enum] -> UnitConverter38/1
  IVI2/19(VHAL_HeadLampSW_enum) -> [VHAL_HeadLampSW_enum]
  UnitConverter39/1 -> bus_creator/42  "VHAL_HeadLampSW_enum"
  [VHAL_HeadLampSW_enum] -> UnitConverter39/1
  IVI2/20(VHAL_HoodLatchSW_enum) -> [VHAL_HoodLatchSW_enum]
  UnitConverter40/1 -> bus_creator/43  "VHAL_HoodLatchSW_enum"
  [VHAL_HoodLatchSW_enum] -> UnitConverter40/1
  IVI2/21(VHAL_IVINightModeSta_flg) -> [VHAL_IVINightModeSta_flg]
  UnitConverter41/1 -> bus_creator/44  "VHAL_IVINightModeSta_flg"
  [VHAL_IVINightModeSta_flg] -> UnitConverter41/1
  IVI2/22(VHAL_IVIPTGModeSW_enum) -> [VHAL_IVIPTGModeSW_enum]
  UnitConverter42/1 -> bus_creator/45  "VHAL_IVIPTGModeSW_enum"
  [VHAL_IVIPTGModeSW_enum] -> UnitConverter42/1
  IVI2/23(VHAL_IVIPTGStaSW_enum) -> [VHAL_IVIPTGStaSW_enum]
  UnitConverter43/1 -> bus_creator/46  "VHAL_IVIPTGStaSW_enum"
  [VHAL_IVIPTGStaSW_enum] -> UnitConverter43/1
  IVI2/24(VHAL_IVIPTGUSStaSW_flg) -> [VHAL_IVIPTGUSStaSW_flg]
  UnitConverter44/1 -> bus_creator/47  "VHAL_IVIPTGUSStaSW_flg"
  [VHAL_IVIPTGUSStaSW_flg] -> UnitConverter44/1
  IVI2/25(VHAL_IVIPWModeReq_enum) -> [VHAL_IVIPWModeReq_enum]
  UnitConverter45/1 -> bus_creator/48  "VHAL_IVIPWModeReq_enum"
  [VHAL_IVIPWModeReq_enum] -> UnitConverter45/1
  IVI2/26(VHAL_IVIPwrLockSW_enum) -> [VHAL_IVIPwrLockSW_enum]
  UnitConverter46/1 -> bus_creator/49  "VHAL_IVIPwrLockSW_enum"
  [VHAL_IVIPwrLockSW_enum] -> UnitConverter46/1
  IVI2/27(VHAL_IVIPwroffreq_flg) -> [VHAL_IVIPwroffreq_flg]
  UnitConverter47/1 -> bus_creator/50  "VHAL_IVIPwroffreq_flg"
  [VHAL_IVIPwroffreq_flg] -> UnitConverter47/1
  IVI2/28(VHAL_IVIRRDefReq_flg) -> [VHAL_IVIRRDefReq_flg]
  UnitConverter48/1 -> bus_creator/51  "VHAL_IVIRRDefReq_flg"
  [VHAL_IVIRRDefReq_flg] -> UnitConverter48/1
  IVI2/29(VHAL_IVIReqV2L_enum) -> [VHAL_IVIReqV2L_enum]
  UnitConverter49/1 -> bus_creator/52  "VHAL_IVIReqV2L_enum"
  [VHAL_IVIReqV2L_enum] -> UnitConverter49/1
  IVI2/30(VHAL_IVIScreen_enum) -> [VHAL_IVIScreen_enum]
  UnitConverter50/1 -> bus_creator/53  "VHAL_IVIScreen_enum"
  [VHAL_IVIScreen_enum] -> UnitConverter50/1
  IVI2/31(VHAL_IVIStartChgreq_flg) -> [VHAL_IVIStartChgreq_flg]
  UnitConverter51/1 -> bus_creator/54  "VHAL_IVIStartChgreq_flg"
  [VHAL_IVIStartChgreq_flg] -> UnitConverter51/1
  IVI2/32(VHAL_IVIStatus_flg) -> [VHAL_IVIStatus_flg]
  UnitConverter52/1 -> bus_creator/55  "VHAL_IVIStatus_flg"
  [VHAL_IVIStatus_flg] -> UnitConverter52/1
  IVI2/33(VHAL_IVIStopChgreq_flg) -> [VHAL_IVIStopChgreq_flg]
  UnitConverter53/1 -> bus_creator/56  "VHAL_IVIStopChgreq_flg"
  [VHAL_IVIStopChgreq_flg] -> UnitConverter53/1
  IVI2/34(VHAL_IVITriggerreq_flg) -> [VHAL_IVITriggerreq_flg]
  UnitConverter54/1 -> bus_creator/57  "VHAL_IVITriggerreq_flg"
  [VHAL_IVITriggerreq_flg] -> UnitConverter54/1
  IVI2/35(VHAL_IVIUnlockChgreq_flg) -> [VHAL_IVIUnlockChgreq_flg]
  UnitConverter55/1 -> bus_creator/58  "VHAL_IVIUnlockChgreq_flg"
  [VHAL_IVIUnlockChgreq_flg] -> UnitConverter55/1
  IVI2/36(VHAL_IVIWIMAINSW_flg) -> [VHAL_IVIWIMAINSW_flg]
  UnitConverter56/1 -> bus_creator/59  "VHAL_IVIWIMAINSW_flg"
  [VHAL_IVIWIMAINSW_flg] -> UnitConverter56/1
  IVI2/37(VHAL_LDrvControlCommand_pct) -> [VHAL_LDrvControlCommand_pct]
  UnitConverter57/1 -> bus_creator/60  "VHAL_LDrvControlCommand_pct"
  [VHAL_LDrvControlCommand_pct] -> UnitConverter57/1
  IVI2/38(VHAL_LPasControlCommand_pct) -> [VHAL_LPasControlCommand_pct]
  UnitConverter58/1 -> bus_creator/61  "VHAL_LPasControlCommand_pct"
  [VHAL_LPasControlCommand_pct] -> UnitConverter58/1
  IVI2/39(VHAL_LRLDControlCommand_pct) -> [VHAL_LRLDControlCommand_pct]
  UnitConverter59/1 -> bus_creator/62  "VHAL_LRLDControlCommand_pct"
  [VHAL_LRLDControlCommand_pct] -> UnitConverter59/1
  IVI2/40(VHAL_LRRDControlCommand_pct) -> [VHAL_LRRDControlCommand_pct]
  UnitConverter60/1 -> bus_creator/63  "VHAL_LRRDControlCommand_pct"
  [VHAL_LRRDControlCommand_pct] -> UnitConverter60/1
  IVI2/41(VHAL_LightShowStartReq_flg) -> [VHAL_LightShowStartReq_flg]
  UnitConverter61/1 -> bus_creator/64  "VHAL_LightShowStartReq_flg"
  [VHAL_LightShowStartReq_flg] -> UnitConverter61/1
  IVI2/42(VHAL_LightShowStopReq_flg) -> [VHAL_LightShowStopReq_flg]
  UnitConverter62/1 -> bus_creator/65  "VHAL_LightShowStopReq_flg"
  [VHAL_LightShowStopReq_flg] -> UnitConverter62/1
  IVI2/43(VHAL_MFRDNBrightReq_pct) -> [VHAL_MFRDNBrightReq_pct]
  UnitConverter63/1 -> bus_creator/66  "VHAL_MFRDNBrightReq_pct"
  [VHAL_MFRDNBrightReq_pct] -> UnitConverter63/1
  IVI2/44(VHAL_OFFACMODE_enum) -> [VHAL_OFFACMODE_enum]
  UnitConverter64/1 -> bus_creator/67  "VHAL_OFFACMODE_enum"
  [VHAL_OFFACMODE_enum] -> UnitConverter64/1
  IVI2/45(VHAL_PSEATventreq_enum) -> [VHAL_PSEATventreq_enum]
  UnitConverter65/1 -> bus_creator/68  "VHAL_PSEATventreq_enum"
  [VHAL_PSEATventreq_enum] -> UnitConverter65/1
  IVI2/46(VHAL_PerdV2L_enum) -> [VHAL_PerdV2L_enum]
  UnitConverter66/1 -> bus_creator/69  "VHAL_PerdV2L_enum"
  [VHAL_PerdV2L_enum] -> UnitConverter66/1
  IVI2/47(VHAL_RFogLampSW_flg) -> [VHAL_RFogLampSW_flg]
  UnitConverter67/1 -> bus_creator/70  "VHAL_RFogLampSW_flg"
  [VHAL_RFogLampSW_flg] -> UnitConverter67/1
  IVI2/48(VHAL_RollModeSWCmd_enum) -> [VHAL_RollModeSWCmd_enum]
  UnitConverter68/1 -> bus_creator/71  "VHAL_RollModeSWCmd_enum"
  [VHAL_RollModeSWCmd_enum] -> UnitConverter68/1
  IVI2/49(VHAL_RoomLampMode_flg) -> [VHAL_RoomLampMode_flg]
  UnitConverter69/1 -> bus_creator/72  "VHAL_RoomLampMode_flg"
  [VHAL_RoomLampMode_flg] -> UnitConverter69/1
  IVI2/50(VHAL_SOCADJBUTT_flg) -> [VHAL_SOCADJBUTT_flg]
  UnitConverter70/1 -> bus_creator/73  "VHAL_SOCADJBUTT_flg"
  [VHAL_SOCADJBUTT_flg] -> UnitConverter70/1
  IVI2/51(VHAL_SOCLimitSet_pct) -> [VHAL_SOCLimitSet_pct]
  UnitConverter71/1 -> bus_creator/74  "VHAL_SOCLimitSet_pct"
  [VHAL_SOCLimitSet_pct] -> UnitConverter71/1
  IVI2/52(VHAL_SOCV2LLimit_pct) -> [VHAL_SOCV2LLimit_pct]
  UnitConverter72/1 -> bus_creator/75  "VHAL_SOCV2LLimit_pct"
  [VHAL_SOCV2LLimit_pct] -> UnitConverter72/1
  IVI2/53(VHAL_SchedChgStart_flg) -> [VHAL_SchedChgStart_flg]
  UnitConverter73/1 -> bus_creator/76  "VHAL_SchedChgStart_flg"
  [VHAL_SchedChgStart_flg] -> UnitConverter73/1
  IVI2/54(VHAL_SchedChgStop_flg) -> [VHAL_SchedChgStop_flg]
  UnitConverter74/1 -> bus_creator/77  "VHAL_SchedChgStop_flg"
  [VHAL_SchedChgStop_flg] -> UnitConverter74/1
  IVI2/55(VHAL_SchedChgbutt_flg) -> [VHAL_SchedChgbutt_flg]
  UnitConverter75/1 -> bus_creator/78  "VHAL_SchedChgbutt_flg"
  [VHAL_SchedChgbutt_flg] -> UnitConverter75/1
  IVI2/56(VHAL_SchedChglimit_pct) -> [VHAL_SchedChglimit_pct]
  UnitConverter76/1 -> bus_creator/79  "VHAL_SchedChglimit_pct"
  [VHAL_SchedChglimit_pct] -> UnitConverter76/1
  IVI2/57(VHAL_SchedChgwake_flg) -> [VHAL_SchedChgwake_flg]
  UnitConverter77/1 -> bus_creator/80  "VHAL_SchedChgwake_flg"
  [VHAL_SchedChgwake_flg] -> UnitConverter77/1
  IVI2/58(VHAL_SenstivityPosition_enum) -> [VHAL_SenstivityPosition_enum]
  UnitConverter78/1 -> bus_creator/81  "VHAL_SenstivityPosition_enum"
  [VHAL_SenstivityPosition_enum] -> UnitConverter78/1
  IVI2/59(VHAL_SetUnlockSingle_flg) -> [VHAL_SetUnlockSingle_flg]
  UnitConverter79/1 -> bus_creator/82  "VHAL_SetUnlockSingle_flg"
  [VHAL_SetUnlockSingle_flg] -> UnitConverter79/1
  IVI2/60(VHAL_TCSSWCmd_enum) -> [VHAL_TCSSWCmd_enum]
  UnitConverter80/1 -> bus_creator/83  "VHAL_TCSSWCmd_enum"
  [VHAL_TCSSWCmd_enum] -> UnitConverter80/1
  IVI2/61(VHAL_TPMSCaliButt_flg) -> [VHAL_TPMSCaliButt_flg]
  UnitConverter81/1 -> bus_creator/84  "VHAL_TPMSCaliButt_flg"
  [VHAL_TPMSCaliButt_flg] -> UnitConverter81/1
  IVI2/62(VHAL_TPMSResButt_flg) -> [VHAL_TPMSResButt_flg]
  UnitConverter82/1 -> bus_creator/85  "VHAL_TPMSResButt_flg"
  [VHAL_TPMSResButt_flg] -> UnitConverter82/1
  IVI2/63(VHAL_TurnSwTimeSet_enum) -> [VHAL_TurnSwTimeSet_enum]
  UnitConverter83/1 -> bus_creator/86  "VHAL_TurnSwTimeSet_enum"
  [VHAL_TurnSwTimeSet_enum] -> UnitConverter83/1
  IVI2/64(VHAL_WalkawayLockSW_flg) -> [VHAL_WalkawayLockSW_flg]
  UnitConverter84/1 -> bus_creator/87  "VHAL_WalkawayLockSW_flg"
  [VHAL_WalkawayLockSW_flg] -> UnitConverter84/1
  IVI2/65(VHAL_WlcmLightMode_enum) -> [VHAL_WlcmLightMode_enum]
  UnitConverter85/1 -> bus_creator/88  "VHAL_WlcmLightMode_enum"
  [VHAL_WlcmLightMode_enum] -> UnitConverter85/1
  IVI2/66(VHAL_sigAirIntenZon1Req_enum) -> [VHAL_sigAirIntenZon1Req_enum]
  UnitConverter86/1 -> bus_creator/89  "VHAL_sigAirIntenZon1Req_enum"
  [VHAL_sigAirIntenZon1Req_enum] -> UnitConverter86/1
  IVI2/67(VHAL_sigDfrstReq_flg) -> [VHAL_sigDfrstReq_flg]
  UnitConverter87/1 -> bus_creator/90  "VHAL_sigDfrstReq_flg"
  [VHAL_sigDfrstReq_flg] -> UnitConverter87/1
  IVI2/68(VHAL_sigFaceReq_flg) -> [VHAL_sigFaceReq_flg]
  UnitConverter88/1 -> bus_creator/91  "VHAL_sigFaceReq_flg"
  [VHAL_sigFaceReq_flg] -> UnitConverter88/1
  IVI2/69(VHAL_sigFootReq_flg) -> [VHAL_sigFootReq_flg]
  UnitConverter89/1 -> bus_creator/92  "VHAL_sigFootReq_flg"
  [VHAL_sigFootReq_flg] -> UnitConverter89/1
  IVI2/70(VHAL_sigRecircReq_flg) -> [VHAL_sigRecircReq_flg]
  UnitConverter90/1 -> bus_creator/93  "VHAL_sigRecircReq_flg"
  [VHAL_sigRecircReq_flg] -> UnitConverter90/1
  IVI2/71(VHAL_sigSetTempZon1Req_C) -> [VHAL_sigSetTempZon1Req_C]
  UnitConverter91/1 -> bus_creator/94  "VHAL_sigSetTempZon1Req_C"
  [VHAL_sigSetTempZon1Req_C] -> UnitConverter91/1
  IVI2/72(VHAL_sigSetTempZon2Req_C) -> [VHAL_sigSetTempZon2Req_C]
  UnitConverter92/1 -> bus_creator/95  "VHAL_sigSetTempZon2Req_C"
  [VHAL_sigSetTempZon2Req_C] -> UnitConverter92/1
  VHAL_CANMsgInvalidIVIP200_flg/1(Out) -> bus_creator/96
  IVI_P20_0/1(VHAL_IVIFrAtmoLampCmd_flg) -> [VHAL_IVIFrAtmoLampCmd_flg]
  UnitConverter93/1 -> bus_creator/97  "VHAL_IVIFrAtmoLampCmd_flg"
  [VHAL_IVIFrAtmoLampCmd_flg] -> UnitConverter93/1
  IVI_P20_0/2(VHAL_IVIPassengerdoorSta_flg) -> [VHAL_IVIPassengerdoorSta_flg]
  UnitConverter94/1 -> bus_creator/98  "VHAL_IVIPassengerdoorSta_flg"
  [VHAL_IVIPassengerdoorSta_flg] -> UnitConverter94/1
  IVI_P20_0/3(VHAL_IVIRrAtmoLampCmd_flg) -> [VHAL_IVIRrAtmoLampCmd_flg]
  UnitConverter95/1 -> bus_creator/99  "VHAL_IVIRrAtmoLampCmd_flg"
  [VHAL_IVIRrAtmoLampCmd_flg] -> UnitConverter95/1
  IVI_P20_0/4(VHAL_IVIRrRmLampBrightCmd_enum) -> [VHAL_IVIRrRmLampBrightCmd_enum]
  UnitConverter96/1 -> bus_creator/100  "VHAL_IVIRrRmLampBrightCmd_enum"
  [VHAL_IVIRrRmLampBrightCmd_enum] -> UnitConverter96/1
  IVI_P20_0/5(VHAL_IVIRrRoomlampCmd_flg) -> [VHAL_IVIRrRoomlampCmd_flg]
  UnitConverter97/1 -> bus_creator/101  "VHAL_IVIRrRoomlampCmd_flg"
  [VHAL_IVIRrRoomlampCmd_flg] -> UnitConverter97/1
  VHAL_CANMsgInvalidMETER1_flg/1(Out) -> bus_creator/102
  METER1/1(VHAL_METERKPHCalcu_kph) -> [VHAL_METERKPHCalcu_kph]
  UnitConverter98/1 -> bus_creator/103  "VHAL_METERKPHCalcu_kph"
  [VHAL_METERKPHCalcu_kph] -> UnitConverter98/1
  METER1/2(VHAL_ODOMETER_km) -> [VHAL_ODOMETER_km]
  UnitConverter99/1 -> bus_creator/104  "VHAL_ODOMETER_km"
  [VHAL_ODOMETER_km] -> UnitConverter99/1
